simulink library "Compression_Air_Water_Chiller"  (Simulink 8.2)
settings: Solver=ode45  StartTime=0.0  StopTime=10.0  RelTol=1e-3
libraries: carnot x3
settings Model: Creator=lena.frank  LastModifiedBy=drhf

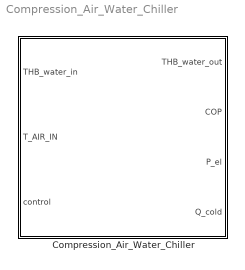
== system Compression_Air_Water_Chiller ==
  Compression_Air_Water_Chiller : Subsystem  mask(compression air/water chiller){Q_Nom=15}
      mask prompts: Q_Nom "Q_Nom [kW]"
      mask help:
      | This block is based on the characteristic curves for cooling capacity and
      | coefficient of performance of the reversible air-to-water heat pump with waste heat recovery LI 16TER+ by Dimplex.
      | The cooling capacity, coefficient of performance, electrical power and THV_WATER_OUT are calculated.
      | The air THV is not calculated due to missing interest.
      | The scaling is based on the point of 11.9 kW.
      |
      | Enter the cooling capacity for the point
      | T_AIR_IN= 30°C, T_WATER_OUT= 7°C.
      | A capacity between 5..50 kW is recommended.
      mask Help: web(fullfile(path_carnot('help'),'compression_chiller.html'),'-helpbrowser')

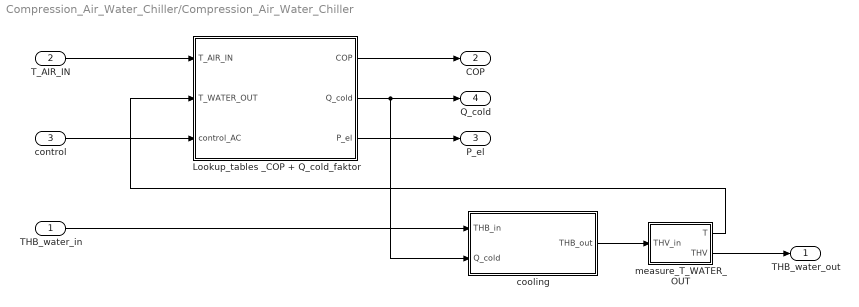
== system Compression_Air_Water_Chiller/Compression_Air_Water_Chiller ==
  THB_water_in : Inport
  T_AIR_IN : Inport  Port=2
  control : Inport  Port=3
  Lookup_tables _COP + Q_cold_faktor : Subsystem  TreatAsAtomicUnit=on
  cooling : Subsystem
  measure_T_WATER_OUT : Subsystem  mask(temperature measurement sensor){tc=10, t0=20}
      mask prompts: tc "time constant of sensor [s]"; t0 "initial temperature [degree centigrade]"
      mask help: Measurement sensor for temperatures with first-oder hold. Temperature is in degree centigrade.
      mask init:
      | tc = 1/max(tc, 0.001);
      mask Help: eval('htmlhelp (''chap_4_2m.htm#measure_T'')')
      mask Display: plot(-18,0,30,20,[0 20],[0 0],[10 10 8 8 12 12 10],[0 8 8 17 17 8 8],[10 10 9 9 11 11 10 9],[15 10 10 9 9 10 9 10])
  THB_water_out : Outport
  COP : Outport  Port=2
  P_el : Outport  Port=3
  Q_cold : Outport  Port=4
  wires:
  Lookup_tables _COP + Q_cold_faktor/1(COP) -> COP/1
  Lookup_tables _COP + Q_cold_faktor/3(P_el) -> P_el/1
  control/1 -> Lookup_tables _COP + Q_cold_faktor/3(control_AC)
  measure_T_WATER_OUT/1(T) -> Lookup_tables _COP + Q_cold_faktor/2(T_WATER_OUT)
  measure_T_WATER_OUT/2(THV) -> THB_water_out/1
  cooling/1(THB_out) -> measure_T_WATER_OUT/1(THV_in)
  T_AIR_IN/1 -> Lookup_tables _COP + Q_cold_faktor/1(T_AIR_IN)
  Lookup_tables _COP + Q_cold_faktor/2(Q_cold) -> Q_cold/1, cooling/2(Q_cold)
  THB_water_in/1 -> cooling/1(THB_in)

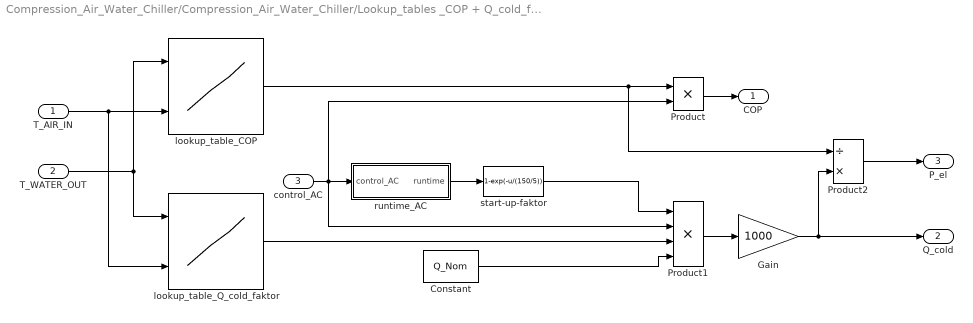
== system Compression_Air_Water_Chiller/Compression_Air_Water_Chiller/Lookup_tables _COP + Q_cold_faktor ==
  T_AIR_IN : Inport
  T_WATER_OUT : Inport  Port=2
  control_AC : Inport  Port=3
  Constant : Constant  Value=Q_Nom
  Gain : Gain  Gain=1000
  Product : Product  RndMeth=Zero
  Product1 : Product  Inputs=4  RndMeth=Zero
  Product2 : Product  Inputs=/*  RndMeth=Zero
  lookup_table_COP : Lookup_n-D  BreakpointsForDimension1=[7,18]  BreakpointsForDimension2=[15,20,25,30,35,40]  BreakpointsForDimension3=[1:2]  BreakpointsForDimension4=[1:2]  Table=[3.55 3.15 2.65 2.25 2 1.7;3.8 3.4 2.93 2.58 2.2 1.95]  InputSameDT=on
  lookup_table_Q_cold_faktor : Lookup_n-D  BreakpointsForDimension1=[7,18]  BreakpointsForDimension2=[15,20,25,30,35,40]  BreakpointsForDimension3=[1:2]  BreakpointsForDimension4=[1:2]  Table=|  InputSameDT=on
      | [ 1.26 1.19 1.08 1.00 0.90 0.79;
      |              1.65 1.53 1.41 1.28 1.18 1.09]
  runtime_AC : Subsystem  TreatAsAtomicUnit=on
      mask help: This block counts the time if input is set to one, it stops counting if input is zero and continues when input rises to one again.
      mask Help: eval('filetest (''manual.htm#count_working_time'')')
  start-up-faktor : Fcn  Expr=1-exp(-u/(150/5))
  COP : Outport
  Q_cold : Outport  Port=2
  P_el : Outport  Port=3
  wires:
  Product2/1 -> P_el/1
  Constant/1 -> Product1/4
  start-up-faktor/1 -> Product1/1
  Product1/1 -> Gain/1
  Product/1 -> COP/1
  runtime_AC/1(runtime) -> start-up-faktor/1
  lookup_table_Q_cold_faktor/1 -> Product1/3
  control_AC/1 -> Product1/2, runtime_AC/1(control_AC), Product/2
  lookup_table_COP/1 -> Product2/1, Product/1
  T_AIR_IN/1 -> lookup_table_COP/2, lookup_table_Q_cold_faktor/2
  T_WATER_OUT/1 -> lookup_table_COP/1, lookup_table_Q_cold_faktor/1
  Gain/1 -> Product2/2, Q_cold/1

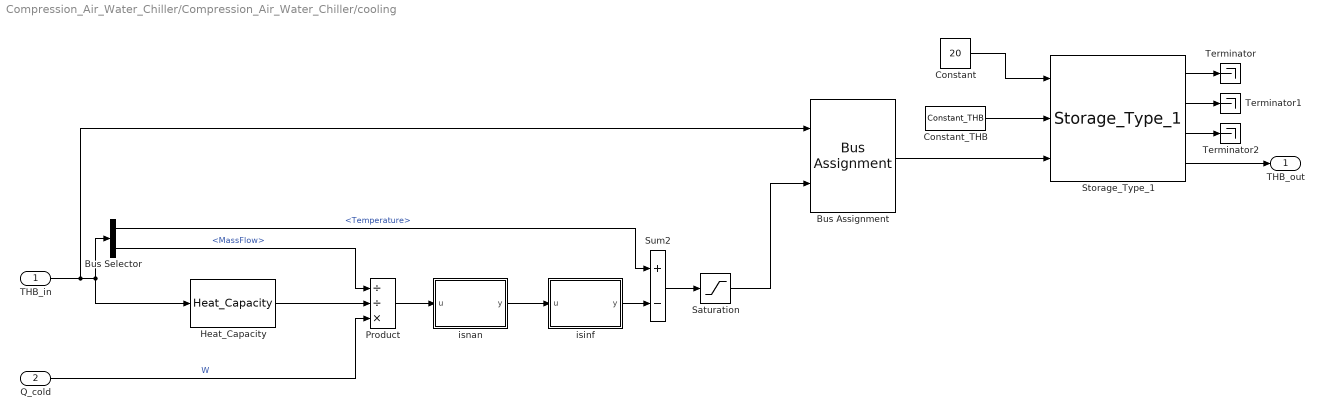
== system Compression_Air_Water_Chiller/Compression_Air_Water_Chiller/cooling ==
  THB_in : Inport
  Q_cold : Inport  Port=2
  Bus Assignment : BusAssignment  AssignedSignals=Temperature
  Bus Selector : BusSelector  OutputSignals=Temperature,MassFlow
  Constant : Constant  Value=20
  Constant_THB : carnot/Source/Simple/Constant_THB  t=40  mdot=0*100/3600  p=1e5  mID=No Pressure Drop  fluid=Water  mix=0  dia=0.02  hgt=0
  Heat_Capacity : carnot/Basic/Material_Properties/Heat_Capacity  VariantControl=CarlibClassic  INPUTARGUMENTS=THB  DEBUGLEVEL=DEBUGLEVEL  MAXTOTALWARNINGS=inf  MAXCONSECUTIVEWARNINGS=inf  WRITETOFILE=0  FILENAME='errors.txt'
  Product : Product  Inputs=//*  SaturateOnIntegerOverflow=on  RndMeth=Zero  InputSameDT=on  OutDataTypeStr=Inherit: Same as first input
  Saturation : Saturate  UpperLimit=inf  LowerLimit=1
  Storage_Type_1 : carnot/Storage/Thermal/Storage_Type_1  uloss=1  ubot=1  utop=1  cond=1  t0=[10:5:55]  volume=0.03  dia=0.01  pos=standing cylinder  nconnect=2  nodes=10  mpoints=10
  Sum2 : Sum  Inputs=+-  InputSameDT=on  OutDataTypeStr=Inherit: Same as first input
  Terminator : Terminator
  Terminator1 : Terminator
  Terminator2 : Terminator
  isinf : MATLAB Function  TreatAsAtomicUnit=on
  isnan : MATLAB Function  TreatAsAtomicUnit=on
  THB_out : Outport
  wires:
  Saturation/1 -> Bus Assignment/2
  Sum2/1 -> Saturation/1
  isinf/1(y) -> Sum2/2
  Product/1 -> isnan/1(u)
  isnan/1(y) -> isinf/1(u)
  Q_cold/1 -> Product/3  "W"
  Bus Selector/1 -> Sum2/1  "<Temperature>"
  THB_in/1 -> Bus Assignment/1, Bus Selector/1, Heat_Capacity/1
  Constant_THB/1 -> Storage_Type_1/2
  Constant/1 -> Storage_Type_1/1
  Bus Assignment/1 -> Storage_Type_1/3
  Heat_Capacity/1 -> Product/2
  Bus Selector/2 -> Product/1  "<MassFlow>"
  Storage_Type_1/4 -> THB_out/1
  Storage_Type_1/1 -> Terminator/1
  Storage_Type_1/2 -> Terminator1/1
  Storage_Type_1/3 -> Terminator2/1

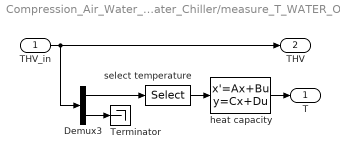
== system Compression_Air_Water_Chiller/Compression_Air_Water_Chiller/measure_T_WATER_OUT ==
  THV_in : Inport
  Demux3 : Demux  Outputs=2
  Terminator : Terminator
  heat capacity : StateSpace  A=-tc  B=tc  D=0  X0=t0
  select temperature : Selector  InputPortWidth=5  IndexOptions=Index vector (dialog)  Indices=[2]  OutputSizes=1
  T : Outport
  THV : Outport  Port=2
  wires:
  heat capacity/1 -> T/1
  select temperature/1 -> heat capacity/1
  THV_in/1 -> THV/1, Demux3/1
  Demux3/1 -> select temperature/1
  Demux3/2 -> Terminator/1

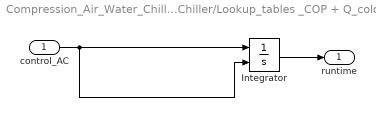
== system Compression_Air_Water_Chiller/Compression_Air_Water_Chiller/Lookup_tables _COP + Q_cold_faktor/runtime_AC ==
  control_AC : Inport
  Integrator : Integrator  ExternalReset=either  InitialCondition=1
  runtime : Outport
  wires:
  Integrator/1 -> runtime/1
  control_AC/1 -> Integrator/1, Integrator/2

== matlab function Compression_Air_Water_Chiller/cooling/isinf ==
  data: u input double; y output double

function y = fcn(u)

% Avoids errors when dividing by very small values. 
% This situation appears when the massflow is near zero.

v = isinf (u);

if v == 0
    
    y = u;

else 
    
    y = 0;
    
end

== matlab function Compression_Air_Water_Chiller/cooling/isnan ==
  data: u input double; y output double

function y = fcn(u)

% Avoids errors when dividing by zero. 
% This situation appears when the massflow is zero.

v = isnan (u);

if v == 0
    
    y = u;

else 
    
    y = 0;
    
end
